simulink model "w3_warplab_buffers"  (Simulink 7.7)
settings: Solver=VariableStepDiscrete  SolverMode=SingleTasking  StartTime=0.0  StopTime=100  RelTol=1e-3
InitFcn:
  | w3_warplab_buffers_init
StartFcn:
  | w3_warplab_buffers_init
values from neighbouring files (symbols this model uses):
  NumSamps_Rx_IQ = 2^15    (= 32768)    [w3_warplab_buffers_init.m]
  NumSamps_Rx_RSSI = 2^13    (= 8192)    [w3_warplab_buffers_init.m]
  NumSamps_Tx_IQ = 2^15    (= 32768)    [w3_warplab_buffers_init.m]
undefined symbols (not defined in the file or in its folder): gcbh, xlBlockLoadCallback, xlGetNormalizedPeriod
libraries: xbsIndex_r4 x453, xbsEDKLib_r4 x1
(part 1 of 5)
settings Model: Creator=mduarte  LastModifiedBy=chunter
settings OptimizationCC: InlineParams=on  InitFltsAndDblsToZero=on
settings DebuggingCC: SaveWithParameterizedLinksMsg=none  StrictBusMsg=Warning
settings GRTTargetCC: TargetFcnLib=ansi_tfl_tmw.mat

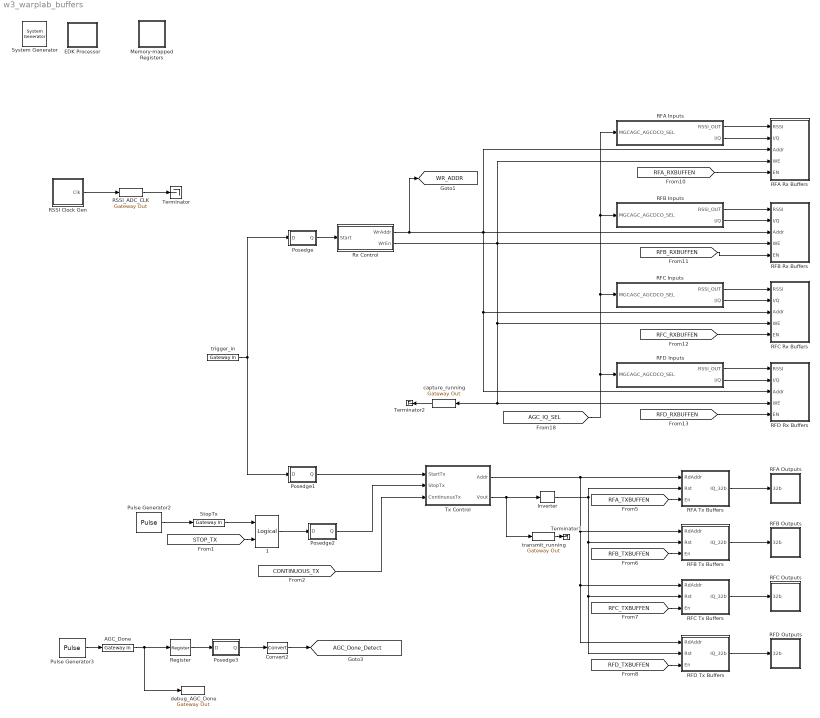
== system w3_warplab_buffers ==
  " 1" : xbsIndex_r4/Logical  logical_function=OR  inputs=2  en=off  latency=0  precision=Full  arith_type=Unsigned  n_bits=16  bin_pt=0  align_bp=on  dbl_ovrd=off  block_type=logical
      settings: block_version=9.1.01
  " System Generator" : xbsIndex_r4/ System Generator  Tag=genX  SystemSampleTime=-1  xilinxfamily=virtex6  part=xc6vlx240t  speed=-2  package=ff1156  synthesis_tool=XST  clock_wrapper=Clock Enables  directory=./netlist  proj_type=Project Navigator  Synth_file=XST Defaults  Impl_file=ISE Defaults  testbench=off  simulink_period=1  sysclk_period=10  dcm_input_clock_period=10  incr_netlist=off  trim_vbits=Everywhere in SubSystem  dbl_ovrd=According to Block Masks  core_generation=According to Block Masks  run_coregen=off  deprecated_control=off  eval_field=0  block_type=sysgen
  AGC_Done : xbsIndex_r4/Gateway In  gui_display_data_type=Fixed-point  arith_type=Unsigned  n_bits=1  bin_pt=0  preci_type=Single  exp_width=8  frac_width=24  quantization="Round  (unbiased: +/- Inf)"  overflow=Saturate  period=1  dbl_ovrd=off  timing_constraint=None  locs_specified=off  LOCs={}  UseAsADC=off  ADCChannel='1'  inherit_from_input=off  hdl_port=on  block_type=gatewayin
      settings: infoedit="Gateway in block.  Converts inputs of type Simulink integer, double and fixed point to  Xilinx fixed point type.<P><P>Hardware notes:  In hardware these blocks become top level input ports."  block_version=VER_STRING_GOES_HERE
  Convert2 : xbsIndex_r4/Convert  gui_display_data_type=Fixed-point  arith_type=Boolean  n_bits=16  bin_pt=14  float_type=Single  exp_bits=8  fraction_bits=24  quantization=Truncate  overflow=Wrap  en=off  latency=0  dbl_ovrd=off  pipeline=off  block_type=convert
      settings: block_version=8.2
  EDK Processor : Subsystem  LoadFcn=xlBlockLoadCallback(gcbh);  mask(Xilinx EDK Processor Block){mode=EDK pcore generation, xmp=, MemVisToProc=<qt bgcolor="#FFFFFF"><div><img src="C:/Xilinx/14.4/ISE_DS/ISE/sysgen/data/images/registerplus.gif"> &lt;&lt;TxDelay&gt;&gt;<br></div><div><img src="C:/Xilinx/14.4/ISE_DS/ISE/sysgen/data/images/registerplus.gif"> &lt;&lt;RX_BUFF_EN&gt;&gt;<br></div><div><img src="C:/Xilinx/14.4/ISE_DS/ISE/sysgen/data/images/registerplus.gif"> &lt;&lt;CONFIG&gt;&gt;<br></div><div><img src="C:/Xilinx/14.4/ISE_DS/ISE/sysgen/data/images/registerplus.gif"> &lt;&lt;TX_BUFF_EN&gt;&gt;<br></div><div><img src="C:/Xilinx/14.4/ISE_DS/ISE/sysgen/data/images/registerplus.gif"> &lt;&lt;BUFF_SIZES&gt;&gt;<br></div><div><img src="C:/Xilinx/14.4/ISE_DS/ISE/sysgen/data/images/registerplus.gif"> &lt;&lt;DESIGN_VER&gt;&gt;<br></div><div><img src="C:/Xilinx/14.4/ISE_DS/ISE/sysgen/data/images/registerplus.gif"> &lt;&lt;STATUS&gt;&gt;<br></div><div><img src="C:/Xilinx/14.4/ISE_DS/ISE/sysgen/data/images/registerplus.gif"> &lt;&lt;RFCD_AGCDoneRSSI&gt;&gt;<br></div><div><img src="C:/Xilinx/14.4/ISE_DS/ISE/sysgen/data/images/registerplus.gif"> &lt;&lt;RFAB_AGCDoneRSSI&gt;&gt;<br></div><div><img src="C:/Xilinx/14.4/ISE_DS/ISE/sysgen/data/images/registerplus.gif"> &lt;&lt;AGCDoneAddr&gt;&gt;<br></div><div><img src="C:/Xilinx/14.4/ISE_DS/ISE/sysgen/data/images/registerplus.gif"> &lt;&lt;RxLength&gt;&gt;<br></div><div><img src="C:/Xilinx/14.4/ISE_DS/ISE/sysgen/data/images/registerplus.gif"> &lt;&lt;TxLength&gt;&gt;<br></div><div><img src="C:/Xilinx/14.4/ISE_DS/ISE/sysgen/data/images/memoryplus.gif"> &lt;&lt;RFD_IQ_Tx_Buffer&gt;&gt;<br></div><div><img src="C:/Xilinx/14.4/ISE_DS/ISE/sysgen/data/images/memoryplus.gif"> &lt;&lt;RFD_RSSI_Buffer&gt;&gt;<br></div><div><img src="C:/Xilinx/14.4/ISE_DS/ISE/sysgen/data/images/memoryplus.gif"> &lt;&lt;RFD_IQ_Rx_Buffer&gt;&gt;<br></div><div><img src="C:/Xilinx/14.4/ISE_DS/ISE/sysgen/data/images/memoryplus.gif"> &lt;&lt;RFC_IQ_Tx_Buffer&gt;&gt;<br></div><div><img src="C:/Xilinx/14.4/ISE_DS/ISE/sysgen/data/images/memoryplus.gif"> &lt;&lt;RFC_RSSI_Buffer&gt;&gt;<br></div><div><img src="C:/Xilinx/14.4/ISE_DS/ISE/sysgen/data/images/memoryplus.gif"> &lt;&lt;RFC_IQ_Rx_Buffer&gt;&gt;<br></div><div><img src="C:/Xilinx/14.4/ISE_DS/ISE/sysgen/data/images/memoryplus.gif"> &lt;&lt;RFB_IQ_Tx_Buffer&gt;&gt;<br></div><div><img src="C:/Xilinx/14.4/ISE_DS/ISE/sysgen/data/images/memoryplus.gif"> &lt;&lt;RFB_RSSI_Buffer&gt;&gt;<br></div><div><img src="C:/Xilinx/14.4/ISE_DS/ISE/sysgen/data/images/memoryplus.gif"> &lt;&lt;RFB_IQ_Rx_Buffer&gt;&gt;<br></div><div><img src="C:/Xilinx/14.4/ISE_DS/ISE/sysgen/data/images/memoryplus.gif"> &lt;&lt;RFA_IQ_Tx_Buffer&gt;&gt;<br></div><div><img src="C:/Xilinx/14.4/ISE_DS/ISE/sysgen/data/images/memoryplus.gif"> &lt;&lt;RFA_RSSI_Buffer&gt;&gt;<br></div><div><img src="C:/Xilinx/14.4/ISE_DS/ISE/sysgen/data/images/memoryplus.gif"> &lt;&lt;RFA_IQ_Rx_Buffer&gt;&gt;<br></div></qt>, AvailableMemories=<empty>, portInterfaceTable={'exposed'=>[],'portdir'=>[],'portname'=>[],'shortname'=>[]}, bus_type_sgadvanced=, bus_type=AXI, baseaddr=0x80000000, baseaddr_lock_sgadvanced=, baseaddr_lock=off, dual_clock_sgadvanced=, dual_clock=on, reg_readback_sgadvanced=, reg_readback=on, ucf_file=, inheritDeviceType_sgadvanced=, inheritDeviceType=off, elf_file=, codebug_sgadvanced=, codebug=on, clock_name=plb, internalPortList={}, resetPolarity=0, memxtable=|, procinfo={}, memmapdirty=off, blockname=, xpsintstyle=default, has_advanced_control=0, sggui_pos=-1,-1,-1,-1, block_type=edkprocessor, block_version=2.7, sg_icon_stat=49,40,-1,-1,white,blue,0,07734,right,,[ ],[ ], sg_mask_display=|, sg_list_contents={'table'=>{'AvailableMemories'=>'popup(<empty>)'}}, sg_blockgui_xml=}
      mask memxtable=|
      | {'mladdr'=>[0.00000000000000000,1.00000000000000000,2.00000000000000000,3.00000000000000000,0.00000000000000000,1.00000000000000000,2.00000000000000000,3.00000000000000000,4.00000000000000000,5.00000000000000000,4.00000000000000000,5.00000000000000000,-1.00000000000000000,-1.00000000000000000,-1.00000000000000000,-1.00000000000000000,-1.00000000000000000,-1.00000000000000000,-1.00000000000000000,-1.00000000000000000,-1.00000000000000000,-1.00000000000000000,-1.00000000000000000,-1.00000000000000000],'mlist'=>['w3_warplab_buffers/Memory-mapped Registers/TxDelay','w3_warplab_buffers/Memory-mapped Registers/From Register16','w3_warplab_buffers/Memory-mapped Registers/From Register13','w3_warplab_buffers/Memory-mapped Registers/From Register1','w3_warplab_buffers/Memory-mapped Registers/To Register3','w3_warplab_buffers/Memory-mapped Registers/To Register2','w3_warplab_buffers/Memory-mapped Registers/To Register1','w3_warplab_buffers/Memory-mapped Registers/Radio3AGCDoneRSSI','w3_warplab_buffers/Memory-mapped Registers/Radio1AGCDoneRSSI','w3_warplab_buffers/Memory-mapped Registers/AGCDoneAddr','w3_warplab_buffers/Memory-mapped Registers/From Register6','w3_warplab_buffers/Memory-mapped Registers/From Register5','w3_warplab_buffers/RFD Tx Buffers/Shared Memory','w3_warplab_buffers/RFD
      | Rx Buffers/RSSI Buffer/Shared Memory','w3_warplab_buffers/RFD
      | Rx Buffers/I//Q Buffer/Shared Memory','w3_warplab_buffers/RFC Tx Buffers/Shared Memory','w3_warplab_buffers/RFC
      | Rx Buffers/RSSI Buffer/Shared Memory','w3_warplab_buffers/RFC
      | Rx Buffers/I//Q Buffer/Shared Memory','w3_warplab_buffers/RFB Tx Buffers/Shared Memory','w3_warplab_buffers/RFB
      | Rx Buffers/RSSI Buffer/Shared Memory','w3_warplab_buffers/RFB
      | Rx Buffers/I//Q Buffer/Shared Memory','w3_warplab_buffers/RFA Tx Buffers/Shared Memory','w3_warplab_buffers/RFA
      | Rx Buffers/RSSI Buffer/Shared Memory','w3_warplab_buffers/RFA
      | Rx Buffers/I//Q Buffer/Shared Memory'],'mlname'=>['\\'TxDelay\\'','\\'RX_BUFF_EN\\'','\\'CONFIG\\'','\\'TX_BUFF_EN\\'','\\'BUFF_SIZES\\'','\\'DESIGN_VER\\'','\\'STATUS\\'','\\'RFCD_AGCDoneRSSI\\'','\\'RFAB_AGCDoneRSSI\\'','\\'AGCDoneAddr\\'','\\'RxLength\\'','\\'TxLength\\'','\\'RFD_IQ_Tx_Buffer\\'','\\'RFD_RSSI_Buffer\\'','\\'RFD_IQ_Rx_Buffer\\'','\\'RFC_IQ_Tx_Buffer\\'','\\'RFC_RSSI_Buffer\\'','\\'RFC_IQ_Rx_Buffer\\'','\\'RFB_IQ_Tx_Buffer\\'','\\'RFB_RSSI_Buffer\\'','\\'RFB_IQ_Rx_Buffer\\'','\\'RFA_IQ_Tx_Buffer\\'','\\'RFA_RSSI_Buffer\\'','\\'RFA_IQ_Rx_Buffer\\''],'mlstate'=>[0.00000000000000000,0.00000000000000000,0.00000000000000000,0.00000000000000000,0.00000000000000000,0.00000000000000000,0.00000000000000000,0.00000000000000000,0.00000000000000000,0.00000000000000000,0.00000000000000000,0.00000000000000000,0.00000000000000000,0.00000000000000000,0.00000000000000000,0.00000000000000000,0.00000000000000000,0.00000000000000000,0.00000000000000000,0.00000000000000000,0.00000000000000000,0.00000000000000000,0.00000000000000000,0.00000000000000000]}
      mask sg_mask_display=|
      | fprintf('','COMMENT: begin icon graphics');
      | patch([0 49 49 0 0 ],[0 0 40 40 0 ],[0.77 0.82 0.91 ]);
      | plot([0 49 49 0 0 ],[0 0 40 40 0 ]);
      | patch([12.875 20.1 25.1 30.1 35.1 25.1 17.875 12.875 ],[25.55 25.55 30.55 25.55 30.55 30.55 30.55 25.55 ],[1 1 1 ]);
      | patch([17.875 25.1 20.1 12.875 17.875 ],[20.55 20.55 25.55 25.55 20.55 ],[0.931 0.946 0.973 ]);
      | patch([12.875 20.1 25.1 17.875 12.875 ],[15.55 15.55 20.55 20.55 15.55 ],[1 1 1 ]);
      | patch([17.875 35.1 30.1 25.1 20.1 12.875 17.875 ],[10.55 10.55 15.55 10.55 15.55 15.55 10.55 ],[0.931 0.946 0.973 ]);
      | fprintf('','COMMENT: end icon graphics');
      | fprintf('','COMMENT: begin icon text');
      | fprintf('','COMMENT: end icon text');
      mask prompts: mode "Configure Processor for"; xmp "XPS Project"; MemVisToProc ""; AvailableMemories "Available Memories"; portInterfaceTable ""; bus_type_sgadvanced ""; bus_type "Bus Type"; baseaddr "Base Address"; baseaddr_lock_sgadvanced ""; baseaddr_lock "Lock"; dual_clock_sgadvanced ""; dual_clock "Dual Clocks"; reg_readback_sgadvanced ""; reg_readback "Register Read-Back"; ucf_file "Constraint File"; inheritDeviceType_sgadvanced ""; inheritDeviceType "Inherit Device Type"; elf_file "Initial Program"; codebug_sgadvanced ""; codebug "Enable Co-Debug with Xilinx SDK (Beta)"; clock_name ""; internalPortList ""; resetPolarity ""; memxtable ""; procinfo ""; memmapdirty ""; blockname ""; xpsintstyle ""; has_advanced_control ""; sggui_pos ""; block_type ""; block_version ""; sg_icon_stat ""; sg_mask_display ""; sg_list_contents ""; sg_blockgui_xml ""
      mask help: Xilinx EDK Processor
      mask init:
      | try
      |   tmp_gcb = gcb;
      |   tmp_gcbh = gcbh;
      |   if (strcmp('SysGenIndex',get_param(bdroot(tmp_gcbh),'tag')) && ~isempty(regexp(bdroot(tmp_gcb), '^xbs', 'once')))
      |     return;
      |   end;
      |   xlMungeMaskParams;
      | 
      |   block_type='edkprocessor';
      | 
      |   serialized_declarations = '{''block_type''=>''String''}';
      |   xledkprocessor_init();
      |   ptable_ = xlblockprep(get_param(tmp_gcb, 'MaskWSVariables'));
      |   try
      |     xlBlockMoveCallback(tmp_gcbh);
      |   catch 
      |      clear global xl_updateicon_recursion_guard;
      |   end;
      | catch
      |   global dbgsysgen;
      |   if(~isempty(dbgsysgen) && dbgsysgen)
      |     e = regexprep(lasterr, '\n', '\nError: ');
      |     disp(['Error: While running MaskInit code on block ' tmp_gcb ': ' e]);
      |     error(e);
      |   end
      | end
      settings: CopyFcn=xlProcBlockCopyCallback(gcbh);xlBlockMoveCallback(gcbh);  DeleteFcn=xlDestroyGui(gcbh);  ModelCloseFcn=xlDestroyGui(gcbh);  PreSaveFcn=xlBlockPreSaveCallback(gcbh);  PostSaveFcn=xlBlockPostSaveCallback(gcbh);  DestroyFcn=xlDestroyGui(gcbh);  OpenFcn=bh=gcbh;xlProcBlockCallbacks('populatesharedmemorylistbox',bh);xlOpenGui(bh, 'edkprocessor_gui.xml', @xlProcBlockEnablement, @xlProcBlockAction);  CloseFcn=xlDestroyGui(gcbh);  MoveFcn=xlBlockMoveCallback(gcbh);
      mask Help: eval('');xlDoc('-book','sysgen','-topic','EDK_Processor');
      mask StyleString: popup(EDK pcore generation|HDL netlisting),edit,edit,edit,edit,edit,popup(AXI|PLB),edit,edit,checkbox,edit,checkbox,edit,checkbox,edit,edit,checkbox,edit,edit,checkbox,edit,edit,edit,edit,edit,edit,edit,edit,edit,edit,edit,edit,edit,edit,edit,edit
      mask Display:
      | fprintf('','COMMENT: begin icon graphics');
      | patch([0 49 49 0 0 ],[0 0 40 40 0 ],[0.77 0.82 0.91 ]);
      | plot([0 49 49 0 0 ],[0 0 40 40 0 ]);
      | patch([12.875 20.1 25.1 30.1 35.1 25.1 17.875 12.875 ],[25.55 25.55 30.55 25.55 30.55 30.55 30.55 25.55 ],[1 1 1 ]);
      | patch([17.875 25.1 20.1 12.875 17.875 ],[20.55 20.55 25.55 25.55 20.55 ],[0.931 0.946 0.973 ]);
      | patch([12.875 20.1 25.1 17.875 12.875 ],[15.55 15.55 20.55 20.55 15.55 ],[1 1 1 ]);
      | patch([17.875 35.1 30.1 25.1 20.1 12.875 17.875 ],[10.55 10.55 15.55 10.55 15.55 15.55 10.55 ],[0.931 0.946 0.973 ]);
      | fprintf('','COMMENT: end icon graphics');
      | fprintf('','COMMENT: begin icon text');
      | disp('');
      | 
      | fprintf('','COMMENT: end icon text');
  Inverter : xbsIndex_r4/Inverter  en=off  latency=0  dbl_ovrd=off  block_type=inv
      settings: block_version=8.2
  Memory-mapped Registers : Subsystem
  Posedge : Subsystem
  Posedge1 : Subsystem
  Posedge2 : Subsystem
  Posedge3 : Subsystem
  Pulse Generator2 : DiscretePulseGenerator  Period=10 * 2^14  PulseWidth=50  PhaseDelay=2.5 * 2^14
  Pulse Generator3 : DiscretePulseGenerator  Period=20000  PulseWidth=50  PhaseDelay=374
  RFA Rx Buffers : Subsystem
  RFA Inputs : Subsystem
  RFA Outputs : Subsystem
  RFA Tx Buffers : Subsystem
  RFB Rx Buffers : Subsystem
  RFB Inputs : Subsystem
  RFB Outputs : Subsystem
  RFB Tx Buffers : Subsystem
  RFC Rx Buffers : Subsystem
  RFC Inputs : Subsystem
  RFC Outputs : Subsystem
  RFC Tx Buffers : Subsystem
  RFD Rx Buffers : Subsystem
  RFD Inputs : Subsystem
  RFD Outputs : Subsystem
  RFD Tx Buffers : Subsystem
  RSSI Clock Gen : Subsystem
  RSSI_ADC_CLK : xbsIndex_r4/Gateway Out  inherit_from_input=off  hdl_port=on  timing_constraint=None  locs_specified=off  LOCs={}  UseAsDAC=off  DACChannel='1'  block_type=gatewayout
      settings: infoedit="Gateway out block.  Converts Xilinx fixed point inputs into ouputs of type Simulink integer, double, or fixed point.<P><P>Hardware notes:  In hardware these blocks become top level output ports or are discarded, depending on how they are configured."  block_version=8.2
  Register : xbsIndex_r4/Register  init=0  rst=off  en=off  dbl_ovrd=off  block_type=register
      settings: block_version=8.2
  Rx Control : Subsystem
  StopTx : xbsIndex_r4/Gateway In  gui_display_data_type=Fixed-point  arith_type=Unsigned  n_bits=1  bin_pt=0  preci_type=Single  exp_width=8  frac_width=24  quantization="Round  (unbiased: +/- Inf)"  overflow=Saturate  period=1  dbl_ovrd=off  timing_constraint=None  locs_specified=off  LOCs={}  UseAsADC=off  ADCChannel='1'  inherit_from_input=off  hdl_port=on  block_type=gatewayin
      settings: infoedit="Gateway in block.  Converts inputs of type Simulink integer, double and fixed point to  Xilinx fixed point type.<P><P>Hardware notes:  In hardware these blocks become top level input ports."  block_version=VER_STRING_GOES_HERE
  Terminator : Terminator
  Terminator1 : Terminator
  Terminator2 : Terminator
  Tx Control : Subsystem
  capture_running : xbsIndex_r4/Gateway Out  inherit_from_input=off  hdl_port=on  timing_constraint=None  locs_specified=off  LOCs={}  UseAsDAC=off  DACChannel='1'  block_type=gatewayout
      settings: infoedit="Gateway out block.  Converts Xilinx fixed point inputs into ouputs of type Simulink integer, double, or fixed point.<P><P>Hardware notes:  In hardware these blocks become top level output ports or are discarded, depending on how they are configured."  block_version=8.2
  debug_AGC_Done : xbsIndex_r4/Gateway Out  inherit_from_input=off  hdl_port=on  timing_constraint=None  locs_specified=off  LOCs={}  UseAsDAC=off  DACChannel='1'  block_type=gatewayout
      settings: infoedit="Gateway out block.  Converts Xilinx fixed point inputs into ouputs of type Simulink integer, double, or fixed point.<P><P>Hardware notes:  In hardware these blocks become top level output ports or are discarded, depending on how they are configured."  block_version=8.2
  transmit_running : xbsIndex_r4/Gateway Out  inherit_from_input=off  hdl_port=on  timing_constraint=None  locs_specified=off  LOCs={}  UseAsDAC=off  DACChannel='1'  block_type=gatewayout
      settings: infoedit="Gateway out block.  Converts Xilinx fixed point inputs into ouputs of type Simulink integer, double, or fixed point.<P><P>Hardware notes:  In hardware these blocks become top level output ports or are discarded, depending on how they are configured."  block_version=8.2
  trigger_in : xbsIndex_r4/Gateway In  gui_display_data_type=Fixed-point  arith_type=Unsigned  n_bits=1  bin_pt=0  preci_type=Single  exp_width=8  frac_width=24  quantization="Round  (unbiased: +/- Inf)"  overflow=Saturate  period=1  dbl_ovrd=off  timing_constraint=None  locs_specified=off  LOCs={}  UseAsADC=off  ADCChannel='1'  inherit_from_input=off  hdl_port=on  block_type=gatewayin
      settings: infoedit="Gateway in block.  Converts inputs of type Simulink integer, double and fixed point to  Xilinx fixed point type.<P><P>Hardware notes:  In hardware these blocks become top level input ports."  block_version=VER_STRING_GOES_HERE
  tag scope: AGC_Done_Detect=global, WR_ADDR=global
  wires:
  [RFC_RXBUFFEN] -> RFC Rx Buffers/5(EN)
  [RFB_RXBUFFEN] -> RFB Rx Buffers/5(EN)
  Posedge/1(Q) -> Rx Control/1(Start)
  RFA Inputs/2(I/Q) -> RFA Rx Buffers/2(I/Q)
  [RFA_RXBUFFEN] -> RFA Rx Buffers/5(EN)
  [RFD_RXBUFFEN] -> RFD Rx Buffers/5(EN)
  Rx Control/1(WrAddr) -> RFB Rx Buffers/3(Addr), RFA Rx Buffers/3(Addr), RFC Rx Buffers/3(Addr), RFD Rx Buffers/3(Addr), [WR_ADDR]
  Rx Control/2(WrEn) -> RFB Rx Buffers/4(WE), RFC Rx Buffers/4(WE), RFD Rx Buffers/4(WE), capture_running/1, RFA Rx Buffers/4(WE)
  RFB Tx Buffers/1(IQ_32b) -> RFB Outputs/1(32b)
  Posedge1/1(Q) -> Tx Control/1(StartTx)
  [CONTINUOUS_TX] -> Tx Control/3(ContinuousTx)
  Posedge2/1(Q) -> Tx Control/2(StopTx)
  " 1"/1 -> Posedge2/1(D)
  StopTx/1 -> " 1"/1
  Pulse Generator2/1 -> StopTx/1
  [RFB_TXBUFFEN] -> RFB Tx Buffers/3(En)
  Tx Control/2(Vout) -> transmit_running/1, Inverter/1
  RFC Tx Buffers/1(IQ_32b) -> RFC Outputs/1(32b)
  [RFC_TXBUFFEN] -> RFC Tx Buffers/3(En)
  RFA Tx Buffers/1(IQ_32b) -> RFA Outputs/1(32b)
  [RFA_TXBUFFEN] -> RFA Tx Buffers/3(En)
  RFD Tx Buffers/1(IQ_32b) -> RFD Outputs/1(32b)
  [RFD_TXBUFFEN] -> RFD Tx Buffers/3(En)
  Tx Control/1(Addr) -> RFC Tx Buffers/1(RdAddr), RFD Tx Buffers/1(RdAddr), RFB Tx Buffers/1(RdAddr), RFA Tx Buffers/1(RdAddr)
  Inverter/1 -> RFC Tx Buffers/2(Rst), RFD Tx Buffers/2(Rst), RFB Tx Buffers/2(Rst), RFA Tx Buffers/2(Rst)
  [STOP_TX] -> " 1"/2
  [AGC_IQ_SEL] -> RFA Inputs/1(MGCAGC_AGCDCO_SEL), RFB Inputs/1(MGCAGC_AGCDCO_SEL), RFC Inputs/1(MGCAGC_AGCDCO_SEL), RFD Inputs/1(MGCAGC_AGCDCO_SEL)
  AGC_Done/1 -> debug_AGC_Done/1, Register/1
  Pulse Generator3/1 -> AGC_Done/1
  Register/1 -> Posedge3/1(D)
  Posedge3/1(Q) -> Convert2/1
  Convert2/1 -> [AGC_Done_Detect]
  capture_running/1 -> Terminator2/1
  transmit_running/1 -> Terminator1/1
  RFA Inputs/1(RSSI_OUT) -> RFA Rx Buffers/1(RSSI)
  RFB Inputs/1(RSSI_OUT) -> RFB Rx Buffers/1(RSSI)
  RFB Inputs/2(I/Q) -> RFB Rx Buffers/2(I/Q)
  RFC Inputs/1(RSSI_OUT) -> RFC Rx Buffers/1(RSSI)
  RFC Inputs/2(I/Q) -> RFC Rx Buffers/2(I/Q)
  RFD Inputs/1(RSSI_OUT) -> RFD Rx Buffers/1(RSSI)
  RFD Inputs/2(I/Q) -> RFD Rx Buffers/2(I/Q)
  trigger_in/1 -> Posedge1/1(D), Posedge/1(D)
  RSSI_ADC_CLK/1 -> Terminator/1
  RSSI Clock Gen/1(Clk) -> RSSI_ADC_CLK/1
